simulink model "rpendtemplate"  (R2016b)
settings: Solver=ode45  StartTime=0.0  StopTime=25  RelTol=1e-3  EnableMultiTasking=on
undefined symbols (not defined in the file or in its folder): adingain, adinoffs, daoutgain, daoutoffs
undefined symbols (not defined in the file): h
settings Model: Creator=rbabuska  LastModifiedBy=wjongeneel
settings DataIOCC: LimitDataPoints=on  SaveFormat=Array  SignalLoggingName=sigsOut
settings OptimizationCC: BooleanDataType=off  ExpressionDepthLimit=2147483647  InitFltsAndDblsToZero=on  LifeSpan=inf
settings DebuggingCC: SaveWithParameterizedLinksMsg=none  SignalResolutionControl=TryResolveAllWithWarning  MultiTaskDSMMsg=warning  MultiTaskCondExecSysMsg=none  AllowSymbolicDim=off  StateNameClashWarn=warning  SFUnexpectedBacktrackingDiag=warning  SFNoUnconditionalDefaultTransitionDiag=warning  SFExecutionAtInitializationDiag=none
settings HardwareCC: ProdBitPerPointer=32  ProdBitPerSizeT=32  ProdBitPerPtrDiffT=32  ProdLargestAtomicFloat=None  ProdIntDivRoundTo=Undefined  ProdEndianess=Unspecified  ProdWordSize=32  ProdHWDeviceType=32-bit Generic  TargetUnknown=on
settings ModelReferenceCC: PropagateSignalLabelsOutOfModel=off
settings GRTTargetCC: TargetFcnLib=ansi_tfl_tmw.mat  TargetLangStandard=C89/C90 (ANSI)  GeneratePreprocessorConditionals=Disable all  CombineOutputUpdateFcns=off  GRTInterface=on
settings ConfigComp: CovMetricSettings=dw  CovHtmlReporting=on  CovSaveCumulativeToWorkspaceVar=on  CovSaveSingleToWorkspaceVar=on  CovExternalEMLEnable=off

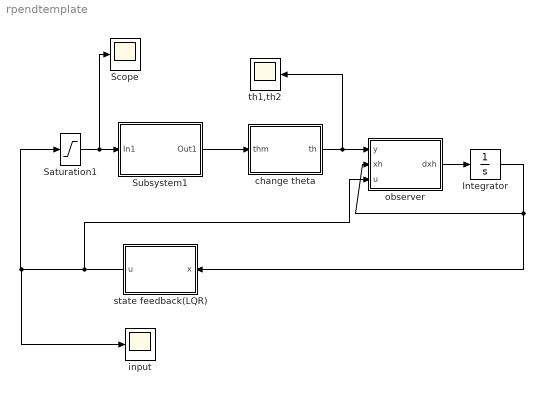
== system rpendtemplate ==
  Integrator : Integrator  InitialCondition=[0;0;0;0;0;0]
  Saturation1 : Saturate  UpperLimit=1  LowerLimit=-1
  Scope : Scope
  Subsystem1 : Subsystem
      mask Display: disp('Rotational\nPendulum')
  change theta : MATLAB Function  TreatAsAtomicUnit=on
  "input " : Scope
  observer : MATLAB Function  TreatAsAtomicUnit=on
  state feedback(LQR) : MATLAB Function  TreatAsAtomicUnit=on
  th1,th2 : Scope
  wires:
  Saturation1/1 -> Scope/1, Subsystem1/1(In1)
  Subsystem1/1(Out1) -> change theta/1(thm)
  change theta/1(th) -> th1,th2/1, observer/1(y)
  observer/1(dxh) -> Integrator/1
  Integrator/1 -> observer/2(xh), state feedback(LQR)/1(x)
  state feedback(LQR)/1(u) -> observer/3(u), Saturation1/1, "input "/1

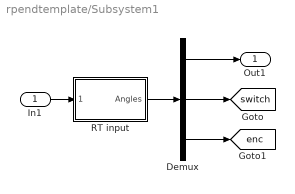
== system rpendtemplate/Subsystem1 ==
  In1 : Inport
  Demux : Demux  Outputs=[2 4 1]
  RT input : Subsystem  mask{Ts=h, channels=[6 7]}
      mask prompts: Ts "Sample time [s]:"; channels "Channels to read (e.g., [6 7])"
      mask init:
      | hwinit;
      | 
      | % initialize FPGA
      | fugihandle = fugiboard('Open', 'Pendulum1');
      | fugihandle.WatchdogTimeout = 0.5;
      | fugiboard('SetParams', fugihandle);
      | fugiboard('Write', fugihandle, 0, 0, 0, 0);  % dummy write to sync interface board
      | fugiboard('Write', fugihandle, 5, 1, 0, 0);  % reset position, activate relay
      | data = fugiboard('Read', fugihandle);        % get version info from FPGA
      | % model = bitshift(data(1), -5); 
      | % version = bitand(data(1), 31);
      | % disp(sprintf('FPGA setup %d, version %d', model, version)); % for the B&P it should say 1 1, or else there is a problem
      | fugiboard('Write', fugihandle, 0, 1, 0, 0);  % end reset
      | pause(0.1);                         % give relay some time to respond
      mask Display: disp('Rotational\nPendulum')
  Out1 : Outport
  tag scope: enc=global, switch=global
  wires:
  RT input/1(Angles) -> Demux/1
  Demux/1 -> Out1/1
  Demux/2 -> [switch]
  Demux/3 -> [enc]
  In1/1 -> RT input/1(Motors)

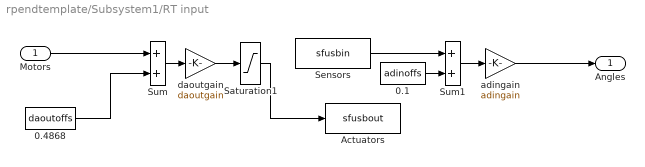
== system rpendtemplate/Subsystem1/RT input ==
  Motors : Inport
  0.1 : Constant  Value=adinoffs
  0.4868 : Constant  Value=daoutoffs
  Actuators : S-Function  FunctionName=sfusbout  Parameters=Ts, fugihandle  SFunctionDeploymentMode=off  EnableBusSupport=off
  Saturation1 : Saturate  UpperLimit=10  LowerLimit=-10
  Sensors : S-Function  FunctionName=sfusbin  Parameters=Ts, fugihandle, channels  SFunctionDeploymentMode=off  EnableBusSupport=off
  Sum : Sum  SaturateOnIntegerOverflow=on  InputSameDT=on  OutDataTypeStr=Inherit: Same as first input
  Sum1 : Sum  SaturateOnIntegerOverflow=on  InputSameDT=on  OutDataTypeStr=Inherit: Same as first input
  adingain : Gain  Gain=adingain  SaturateOnIntegerOverflow=on  OutDataTypeStr=Inherit: Same as input  ParamDataTypeStr=Inherit: Same as input
  daoutgain : Gain  Gain=daoutgain  SaturateOnIntegerOverflow=on  OutDataTypeStr=Inherit: Same as input  ParamDataTypeStr=Inherit: Same as input
  Angles : Outport
  wires:
  Sum/1 -> daoutgain/1
  0.4868/1 -> Sum/2
  Motors/1 -> Sum/1
  Sum1/1 -> adingain/1
  0.1/1 -> Sum1/2
  Sensors/1 -> Sum1/1
  adingain/1 -> Angles/1
  Saturation1/1 -> Actuators/1
  daoutgain/1 -> Saturation1/1

== matlab function rpendtemplate/state feedback(LQR) ==
  data: x input; u output
function u = K(x)
K = [-0.9881 -25.5096 -1.3137 -2.5503 0.7927 10.1199];
u = -K*x;

== matlab function rpendtemplate/change theta ==
  data: thm input; th output
function th = changeOfCoords(thm)
% change the measurements towards our coordinate system 
th = zeros(2,1);
th(1) = pi/2-thm(1);
th(2) = th(1)-thm(2);
% we control around up,up, thus
th(1) = th(1)-pi/2;
th(2) = th(2)-pi/2;

== matlab function rpendtemplate/observer ==
  data: y input; dxh output; xh input; u input
function dxh = obs(y,xh,u)

Ae = 1.0e+03*[0         0    0.0010         0         0         0;
         0         0         0    0.0010         0         0;
    0.0044   -0.0011   -0.0238    0.0000   -1.1953    5.2197;
   -0.0047    0.1077    0.0259   -0.0012    1.2993   -5.6740;
         0         0         0         0   -0.0531   -0.1589;
         0         0         0         0    0.3349   -0.3018];
Ce =[1 0 0 0 0 0;
    0 1 0 0 0  0]; 
Be =    [0;
         0;
         0;
         0;
  -21.2530;
   82.6779];
L =    1.0e+04*[0.0138    0.0068   -0.5930    1.7270    0.0279    0.0651
    0.0105    0.0085    1.8364   -0.9924   -0.0347   -0.1266]; 
yh = Ce*xh;
dxh = Ae*xh+Be*u+L'*(y-yh);
